simulink model "First_Second_OrderSystems"  (R2023b)
settings: Solver=FixedStepAuto  StartTime=0.0  StopTime=10.0  FixedStep=1e-3  RelTol=1e-3
settings Model: Creator=MOHAMED  LastModifiedBy=MOHAMED

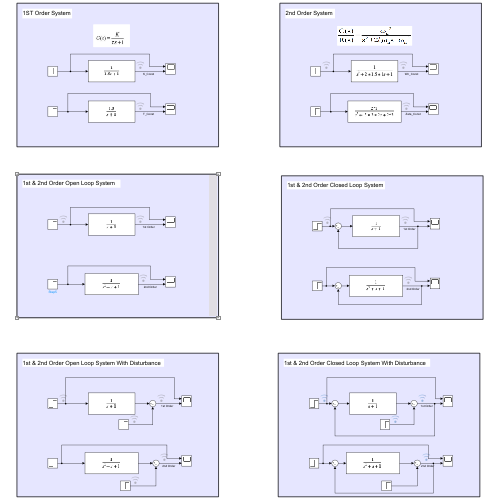
[thumbnail: Simulink's stored preview of the top-level diagram]
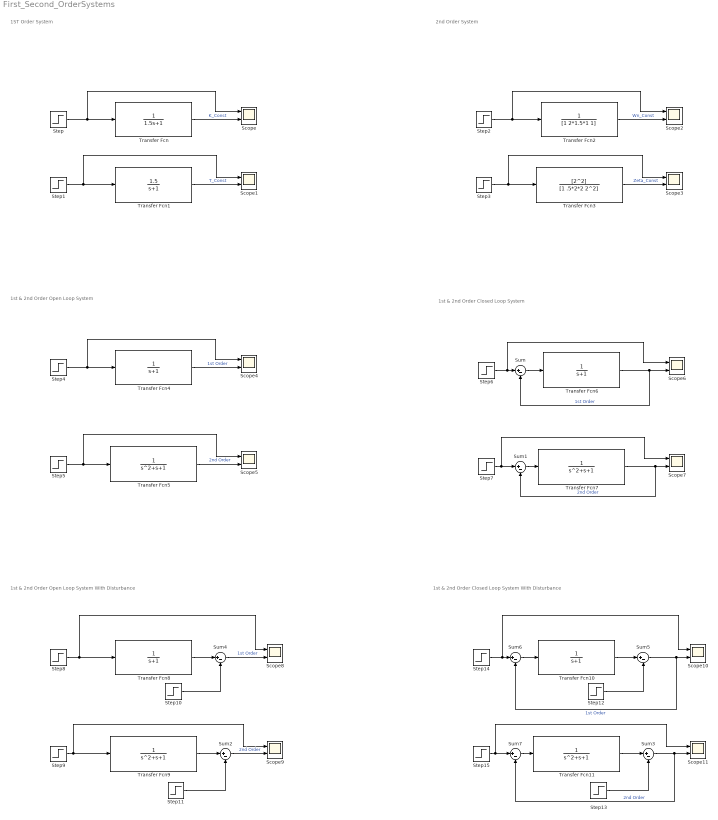
== system First_Second_OrderSystems ==
  note: 1ST Order System
  note: 2nd Order System
  note: 1st & 2nd Order Open Loop System
  note: 1st & 2nd Order Closed Loop System
  note: 1st & 2nd Order Open Loop System With Disturbance
  note: 1st & 2nd Order Closed Loop System With Disturbance
  Scope{,1..11} (12 alike) : Scope  NumInputPorts=2
  Step{,1..9,14..15} (12 alike) : Step  SampleTime=0
  Step{10..13} (4 alike) : Step  Time=3  After=0.5  SampleTime=0
  Sum{,1..7} (8 alike) : Sum  Inputs=|+-
  Transfer Fcn : TransferFcn  Denominator=[1.5 1]
  Transfer Fcn1 : TransferFcn  Numerator=[1.5]  Denominator=[1 1]
  Transfer Fcn{4,6,8,10} (4 alike) : TransferFcn  Denominator=[1 1]
  Transfer Fcn{5,7,9,11} (4 alike) : TransferFcn  Denominator=[1 1 1]
  Transfer Fcn2 : TransferFcn  Denominator=[1 2*1.5*1 1]
  Transfer Fcn3 : TransferFcn  Numerator=[2^2]  Denominator=[1 .5*2*2 2^2]
  wires:
  Step/1 -> Scope/1, Transfer Fcn/1
  Transfer Fcn/1 -> Scope/2  "K_Const"
  Transfer Fcn1/1 -> Scope1/2  "T_Const"
  Step1/1 -> Scope1/1, Transfer Fcn1/1
  Step3/1 -> Transfer Fcn3/1, Scope3/1
  Transfer Fcn3/1 -> Scope3/2  "Zeta_Const"
  Transfer Fcn2/1 -> Scope2/2  "Wn_Const"
  Step2/1 -> Transfer Fcn2/1, Scope2/1
  Step4/1 -> Scope4/1, Transfer Fcn4/1
  Transfer Fcn4/1 -> Scope4/2  "1st Order"
  Transfer Fcn5/1 -> Scope5/2  "2nd Order"
  Step5/1 -> Scope5/1, Transfer Fcn5/1
  Step7/1 -> Sum1/1, Scope7/1
  Transfer Fcn7/1 -> Sum1/2, Scope7/2  "2nd Order"
  Transfer Fcn6/1 -> Scope6/2, Sum/2  "1st Order"
  Step6/1 -> Sum/1, Scope6/1
  Sum/1 -> Transfer Fcn6/1
  Sum1/1 -> Transfer Fcn7/1
  Step9/1 -> Transfer Fcn9/1, Scope9/1
  Step8/1 -> Scope8/1, Transfer Fcn8/1
  Transfer Fcn8/1 -> Sum4/1
  Sum4/1 -> Scope8/2  "1st Order"
  Step10/1 -> Sum4/2
  Transfer Fcn9/1 -> Sum2/1
  Step11/1 -> Sum2/2
  Sum2/1 -> Scope9/2  "2nd Order"
  Sum3/1 -> Sum7/2, Scope11/2  "2nd Order"
  Step13/1 -> Sum3/2
  Transfer Fcn11/1 -> Sum3/1
  Step12/1 -> Sum5/2
  Sum5/1 -> Scope10/2, Sum6/2  "1st Order"
  Transfer Fcn10/1 -> Sum5/1
  Step14/1 -> Sum6/1, Scope10/1
  Step15/1 -> Sum7/1, Scope11/1
  Sum6/1 -> Transfer Fcn10/1
  Sum7/1 -> Transfer Fcn11/1
